simulink model "Prac3_setup_R2019b"  (R2019b)
settings: Solver=VariableStepAuto  StartTime=0.0  StopTime=10  RelTol=1e-3
values from neighbouring files (symbols this model uses):
  A = [0 1 ... (first row only)    [Practical3.m]
  B = [ 0 ... (first row only)    [Practical3.m]
  C = [b2 0]    [Practical3.m]
  K = [16^2-a2  16-a1]    [Practical3.m]
  M = [m1;m2]    [Practical3.m]
  N = -1/(C*inv(A-B*K)*B)    [Practical3.m]
  prac3_param1 = 10.0595705167    [Prac3_paramaters007.mat]
  prac3_param2 = 0.01    [Prac3_paramaters007.mat]
  prac3_param3 = 0.17097230168    [Prac3_paramaters007.mat]
  prac3_param4 = 100    [Prac3_paramaters007.mat]
  prac3_param5 = 0.845451626268    [Prac3_paramaters007.mat]
  prac3_param6 = 0.01    [Prac3_paramaters007.mat]
settings Model: Creator=mluser  LastModifiedBy=waltd

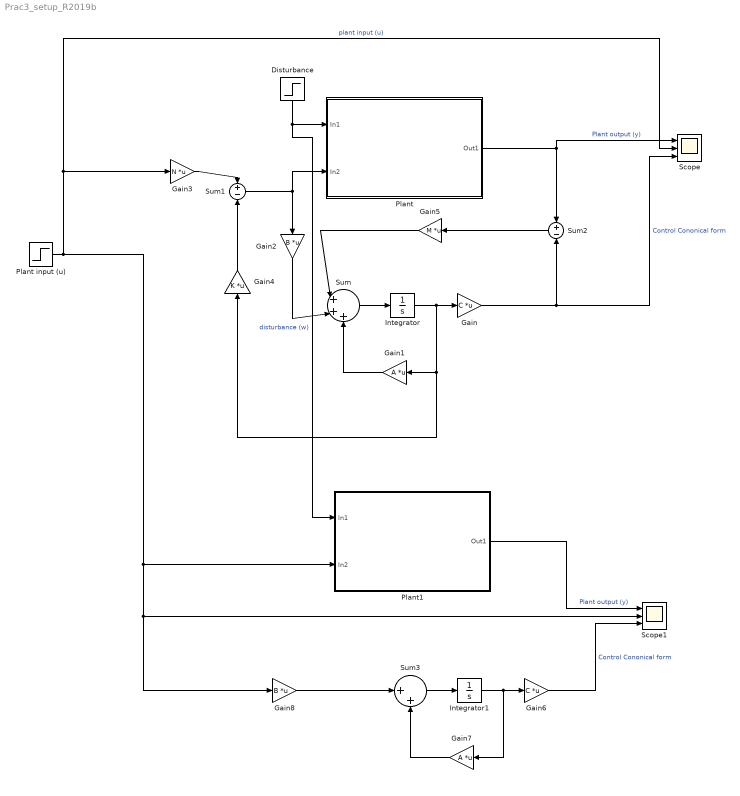
== system Prac3_setup_R2019b ==
  Disturbance : Step  Time=5  After=0  SampleTime=0
  Gain : Gain  Gain=C  Multiplication=Matrix(K*u)
  Gain1 : Gain  Gain=A  Multiplication=Matrix(K*u)
  Gain2 : Gain  Gain=B  Multiplication=Matrix(K*u)
  Gain3 : Gain  Gain=N  Multiplication=Matrix(K*u)
  Gain4 : Gain  Gain=K  Multiplication=Matrix(K*u)
  Gain5 : Gain  Gain=M  Multiplication=Matrix(K*u)
  Gain6 : Gain  Gain=C  Multiplication=Matrix(K*u)
  Gain7 : Gain  Gain=A  Multiplication=Matrix(K*u)
  Gain8 : Gain  Gain=B  Multiplication=Matrix(K*u)
  Integrator : Integrator
  Integrator1 : Integrator
  Plant : Subsystem
  Plant input (u) : Step  SampleTime=0
  Plant1 : Subsystem
  Scope : Scope  NumInputPorts=3
  Scope1 : Scope  NumInputPorts=3
  Sum : Sum  Inputs=|+++
  Sum1 : Sum  Inputs=+-
  Sum2 : Sum  Inputs=+-
  Sum3 : Sum  Inputs=|++
  wires:
  Disturbance/1 -> Plant1/1(In1), Plant/1(In1)  "disturbance (w)"
  Plant/1(Out1) -> Scope/1, Sum2/1  "Plant output (y)"
  Sum/1 -> Integrator/1
  Gain/1 -> Sum2/2, Scope/3  "Control Cononical form"
  Gain1/1 -> Sum/3
  Gain2/1 -> Sum/2
  Plant input (u)/1 -> Plant1/2(In2), Scope1/2, Gain8/1, Gain3/1, Scope/2  "plant input (u)"
  Sum1/1 -> Plant/2(In2), Gain2/1
  Gain3/1 -> Sum1/1
  Gain4/1 -> Sum1/2
  Sum2/1 -> Gain5/1
  Integrator/1 -> Gain1/1, Gain4/1, Gain/1
  Gain5/1 -> Sum/1
  Sum3/1 -> Integrator1/1
  Integrator1/1 -> Gain7/1, Gain6/1
  Gain7/1 -> Sum3/2
  Gain6/1 -> Scope1/3  "Control Cononical form"
  Gain8/1 -> Sum3/1
  Plant1/1(Out1) -> Scope1/1  "Plant output (y)"

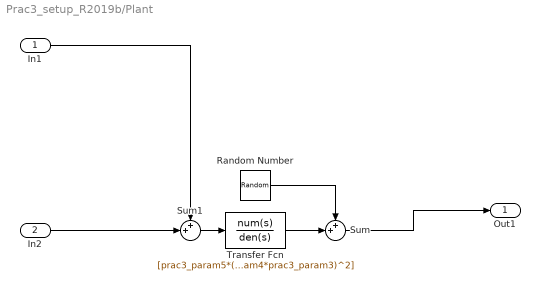
== system Prac3_setup_R2019b/Plant ==
  In1 : Inport
  In2 : Inport  Port=2
  Random Number : RandomNumber  Variance=prac3_param6^2  SampleTime=0.001
  Sum : Sum  Inputs=++|
  Sum1 : Sum  Inputs=++|
  Transfer Fcn : TransferFcn  Numerator=[prac3_param5*(prac3_param4*prac3_param3)^2]  Denominator=[1 2*prac3_param4*prac3_param3*prac3_param2*prac3_param1 (prac3_param4*prac3_param3)^2]
  Out1 : Outport
  wires:
  Sum/1 -> Out1/1
  Transfer Fcn/1 -> Sum/2
  In2/1 -> Sum1/2
  In1/1 -> Sum1/1
  Sum1/1 -> Transfer Fcn/1
  Random Number/1 -> Sum/1

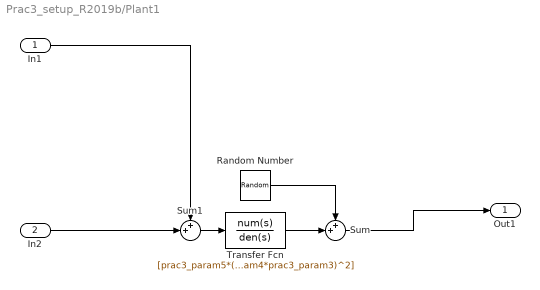
== system Prac3_setup_R2019b/Plant1 ==
  In1 : Inport
  In2 : Inport  Port=2
  Random Number : RandomNumber  Variance=prac3_param6^2  SampleTime=0.001
  Sum : Sum  Inputs=++|
  Sum1 : Sum  Inputs=++|
  Transfer Fcn : TransferFcn  Numerator=[prac3_param5*(prac3_param4*prac3_param3)^2]  Denominator=[1 2*prac3_param4*prac3_param3*prac3_param2*prac3_param1 (prac3_param4*prac3_param3)^2]
  Out1 : Outport
  wires:
  Sum/1 -> Out1/1
  Transfer Fcn/1 -> Sum/2
  In2/1 -> Sum1/2
  In1/1 -> Sum1/1
  Sum1/1 -> Transfer Fcn/1
  Random Number/1 -> Sum/1
